simulink model "URPAAnalyser"  (R2021a)
settings: Solver=FixedStepAuto  StartTime=0.0  StopTime=5.0  RelTol=1e-3  EnableMultiTasking=on
values from neighbouring files (symbols this model uses):
  c = 1.397    [TonAnalyzer.m]
  fcoefs = MakeERBFilters(22050,64,100)    [ERBFilterBank.m]
  imH = imag(H)    [URPAAnalyzer.m]
  imH16k = imag(H16k)    [URPAAnalyzer.m]
  reH = real(H)    [URPAAnalyzer.m]
  reH16k = real(H16k)    [URPAAnalyzer.m]
  xr = xr(:)'    [URPAAnalyzer.m]
undefined symbols (not defined in the file or in its folder): a, b, d, fsam, gzi, Nch
settings Model: Creator=Jaume Segura  LastModifiedBy=Jaume Segura
settings SolverCC: PositivePriorityOrder=on
settings OptimizationCC: EnhancedBackFolding=on  PassReuseOutputArgsAs=Individual arguments  ZeroExternalMemoryAtStartup=off  ZeroInternalMemoryAtStartup=off  MaxStackSize=64  OptimizeBlockOrder=speed  DifferentSizesBufferReuse=on  OptimizationCustomize=off  EfficientTunableParamExpr=on
settings DebuggingCC: ParameterTunabilityLossMsg=error
settings HardwareCC: ProdBitPerPointer=32  ProdBitPerSizeT=32  ProdBitPerPtrDiffT=32  ProdLargestAtomicInteger=Long  ProdLargestAtomicFloat=Double  ProdWordSize=32  ProdLongLongMode=on  ProdHWDeviceType=ARM Compatible->ARM Cortex
settings RTWCC: SystemTargetFile=ert.tlc  HardwareBoard=Raspberry Pi  TLCOptions="-aInlineSetEventsForThisBaseRateFcn=TLC_FALSE -aSuppressMultiTaskScheduler=TLC_FALSE  -aRateBasedStepFcn=0"  TemplateMakefile=ert_default_tmf  Toolchain=GNU GCC Embedded Linux  BuildConfiguration=Faster Runs
settings CodeAppCC: ForceParamTrailComments=on  IgnoreCustomStorageClasses=off  OperatorAnnotations=on  SimulinkDataObjDesc=on  SFDataObjDesc=on  InsertBlockDesc=on
settings ERTTargetCC: SupportVariableSizeSignals=on  ExtModeTransport=2  ExtModeStaticAlloc=on  ExtModeMexFile=ext_xcp  ExtModeIntrfLevel=Level2 - Open

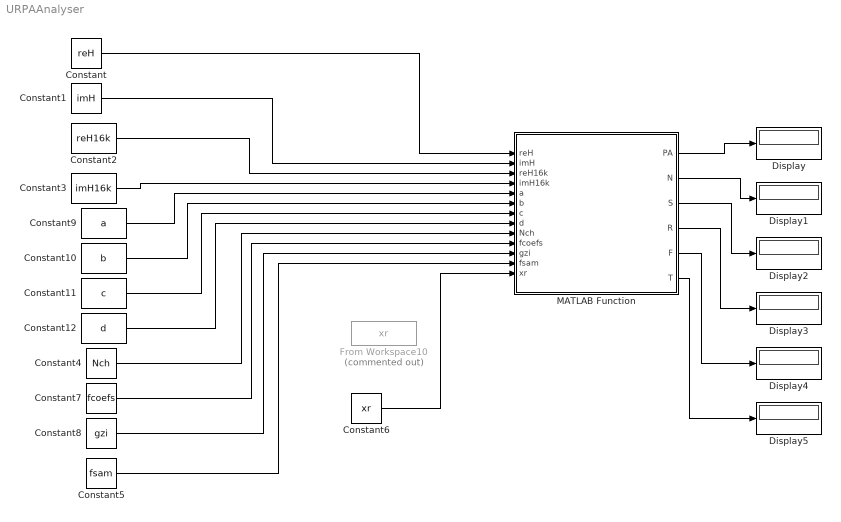
== system URPAAnalyser ==
  Constant : Constant  Value=reH
  Constant1 : Constant  Value=imH
  Constant10 : Constant  Value=b
  Constant11 : Constant  Value=c
  Constant12 : Constant  Value=d
  Constant2 : Constant  Value=reH16k
  Constant3 : Constant  Value=imH16k
  Constant4 : Constant  Value=Nch
  Constant5 : Constant  Value=fsam
  Constant6 : Constant  Value=xr
  Constant7 : Constant  Value=fcoefs
  Constant8 : Constant  Value=gzi
  Constant9 : Constant  Value=a
  Display{,1..5} (6 alike) : Display
  From Workspace10 : FromWorkspace  Commented=on  VariableName=xr
  MATLAB Function : MATLAB Function  TreatAsAtomicUnit=on
  wires:
  Constant5/1 -> MATLAB Function/12(fsam)
  MATLAB Function/1(PA) -> Display/1
  MATLAB Function/6(T) -> Display5/1
  MATLAB Function/2(N) -> Display1/1
  Constant12/1 -> MATLAB Function/8(d)
  Constant9/1 -> MATLAB Function/5(a)
  Constant10/1 -> MATLAB Function/6(b)
  Constant8/1 -> MATLAB Function/11(gzi)
  Constant7/1 -> MATLAB Function/10(fcoefs)
  Constant6/1 -> MATLAB Function/13(xr)
  Constant1/1 -> MATLAB Function/2(imH)
  Constant2/1 -> MATLAB Function/3(reH16k)
  Constant3/1 -> MATLAB Function/4(imH16k)
  Constant/1 -> MATLAB Function/1(reH)
  Constant4/1 -> MATLAB Function/9(Nch)
  MATLAB Function/5(F) -> Display4/1
  Constant11/1 -> MATLAB Function/7(c)
  MATLAB Function/4(R) -> Display3/1
  MATLAB Function/3(S) -> Display2/1

== matlab function URPAAnalyser/MATLAB Function ==
  data: PA output; N output; S output; R output; F output; reH input; imH input; reH16k input; imH16k input; a input; b input; c input; d input; Nch input; fcoefs input; gzi input; fsam input; xr input; T output
function [PA,N,S,R,F,T]= URPAAnalyzer(reH,imH, reH16k,imH16k,a,b,c,d,Nch,fcoefs,gzi,fsam,xr) %%%%%%%%%#codegen

    %H=reH+1i*imH;
    %H16k=reH16k+1i*imH16k;
    
    %addpath('libraries');
    %addpath('libraries\libNS');
    %addpath('libraries\libR');
    %addpath('libraries\libF');
    %addpath('libraries\libTon');
    
    % Create a Raspberry Pi object
    %r= raspi();
    %fsam=double(0);
    %audioFile='highPAsound.wav';
    %[xr,fsam] = audioread(audioFile);
    if(size(xr,1)==1)
        xr=xr';
    end
    
    %fsam=44100;
    fs = 16000;
    if (fsam ~= fs)
        xs = resample1(xr,fs,fsam);
    else
        xs = xr;
    end
    
    N=double(0);
    S=double(0);
    R=double(0);
    F=double(0);
    T=double(0);
    
    %tic
    [N, S] = NSAnalyzer(xs,reH,imH,fs);
    R = RAnalyzer(xs,a,b,c,d,Nch,fcoefs,gzi,fs);
    F = FAnalyzer(xs,b,a,d,c,Nch,fcoefs,gzi,fs);
%
%  G.-Q. Di, X.-W. Chen, K. Song, B. Zhou,Ch.-M. Pei, "Improvement of Zwicker’s psychoacoustic annoyance model aiming at tonal noises".
%  Applied Acoustics 105 (2016) pp.164–170
    [T,~,~,~,~]=TonAnalyzer(xr,fs,reH16k,imH16k);

    wS=double(0);
    wFR=double(0);
    wT=double(0);

    wS = (S-1.75).* 0.25 .* log10(N+10);
    wFR = (2.18 ./ (N.^0.4)) .* ((0.4.*F) + (0.6 .* R)); 
    wT = (6.41./(N.^0.52))*T;
    if (T>=0.3)
        PA = N .* (1 + sqrt((wS.^2) + (wFR.^2) + (wT.^2)));
    else
        PA = N .* (1 + sqrt((wS.^2) + (wFR.^2)));
    end
    %toc

end
